simulink model "open_loop"  (R2021b)
settings: Solver=VariableStepAuto  StartTime=0.0  StopTime=100.0  RelTol=1e-3
values from neighbouring files (symbols this model uses):
  A = zeros(size(B'))    [parameters.m]
  I = 4000*eye(3)    [parameters.m]
  Iz = I(end)    [particle_mpc.m]
  m = length(arch_type)    [batch_simulation.m]    (also in particle_mpc.m = mass)
  mass = 2000    [parameters.m]
  r_1 = [front_length;width/2;-height]    [parameters.m]
  radius = 0.4    [parameters.m]
  rear_length = 1.6    [parameters.m]
  sys_d = c2d(sys, ts)    [particle_mpc.m]
  ts = 0.5    [particle_mpc.m]
libraries: nesl_utility x9, autolibshared x5, vrlib x4, mpclib x1
(part 4 of 4)

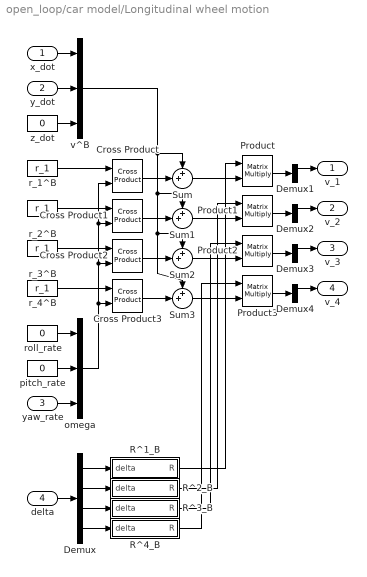
== system open_loop/car model/Longitudinal wheel motion ==
  x_dot : Inport
  y_dot : Inport  Port=2
  yaw_rate : Inport  Port=3
  delta : Inport  Port=4
  Cross Product{,1..3} (4 alike) : vrlib/Utilities/Cross Product
  Demux : Demux
  Demux{1..4} (4 alike) : Demux  Outputs=3
  Product{,1..3} (4 alike) : Product  Multiplication=Matrix(*)
  R^1_B : MATLAB Function  TreatAsAtomicUnit=on
  R^2_B : MATLAB Function  TreatAsAtomicUnit=on
  R^3_B : MATLAB Function  TreatAsAtomicUnit=on
  R^4_B : MATLAB Function  TreatAsAtomicUnit=on
  Sum{,1..3} (4 alike) : Sum  Inputs=++|
  omega : Mux  Inputs=3
  pitch_rate : Constant  Value=0
  r_1^B : Constant  Value=r_1
  r_2^B : Constant  Value=r_1
  r_3^B : Constant  Value=r_1
  r_4^B : Constant  Value=r_1
  roll_rate : Constant  Value=0
  v^B : Mux  Inputs=3
  z_dot : Constant  Value=0
  v_1 : Outport
  v_2 : Outport  Port=2
  v_3 : Outport  Port=3
  v_4 : Outport  Port=4
  wires:
  x_dot/1 -> v^B/1
  y_dot/1 -> v^B/2
  z_dot/1 -> v^B/3
  yaw_rate/1 -> omega/3
  roll_rate/1 -> omega/1
  pitch_rate/1 -> omega/2
  r_1^B/1 -> Cross Product/1
  omega/1 -> Cross Product3/2, Cross Product2/2, Cross Product/2, Cross Product1/2
  r_2^B/1 -> Cross Product1/1
  r_3^B/1 -> Cross Product2/1
  r_4^B/1 -> Cross Product3/1
  Cross Product/1 -> Sum/2
  Cross Product1/1 -> Sum1/2
  Cross Product2/1 -> Sum2/2
  Cross Product3/1 -> Sum3/2
  v^B/1 -> Sum/1, Sum1/1, Sum2/1, Sum3/1
  delta/1 -> Demux/1
  Demux/1 -> R^1_B/1(delta)
  Demux/2 -> R^2_B/1(delta)
  Demux/3 -> R^3_B/1(delta)
  Demux/4 -> R^4_B/1(delta)
  Sum/1 -> Product/2
  Sum1/1 -> Product1/2
  Sum2/1 -> Product2/2
  Sum3/1 -> Product3/2
  R^1_B/1(R) -> Product/1
  R^2_B/1(R) -> Product1/1
  R^3_B/1(R) -> Product2/1
  R^4_B/1(R) -> Product3/1
  Product/1 -> Demux1/1
  Demux1/1 -> v_1/1
  Demux2/1 -> v_2/1
  Demux3/1 -> v_3/1
  Demux4/1 -> v_4/1
  Product3/1 -> Demux4/1
  Product1/1 -> Demux2/1
  Product2/1 -> Demux3/1

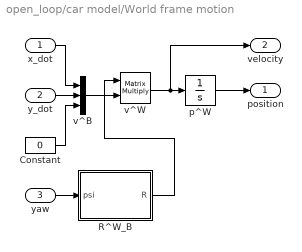
== system open_loop/car model/World frame motion ==
  x_dot : Inport
  y_dot : Inport  Port=2
  yaw : Inport  Port=3
  Constant : Constant  Value=0
  R^W_B : MATLAB Function  TreatAsAtomicUnit=on
  p^W : Integrator
  v^B : Mux  Inputs=3
  v^W : Product  Multiplication=Matrix(*)
  position : Outport
  velocity : Outport  Port=2
  wires:
  yaw/1 -> R^W_B/1(psi)
  y_dot/1 -> v^B/2
  x_dot/1 -> v^B/1
  Constant/1 -> v^B/3
  v^B/1 -> v^W/2
  R^W_B/1(R) -> v^W/1
  v^W/1 -> velocity/1, p^W/1
  p^W/1 -> position/1

== matlab function open_loop/car model/Longitudinal wheel motion/R^1_B ==
  data: delta input; R output
function R = wheel_rotation(delta)
R=[cos(delta) sin(delta) 0
  -sin(delta) cos(delta) 0
  0 0 1];

== matlab function open_loop/MPC/MATLAB Function ==
  data: u input; state input; output input; B output; X output; Y output; U output; DX output; m input; Iz input; Ts input
function [B, X, Y, U, DX] = fcn(u, state, output, m, Iz, Ts)
    A_c = [0 0 0 1 0 0;
     0 0 0 0 1 0;
     0 0 0 0 0 1;
     0 0 0 0 0 0;
     0 0 0 0 0 0;
     0 0 0 0 0 0];
    B = [zeros(3,3); 
          [cos(output(3))/m -sin(output(3))/m 0;
           sin(output(3))/m  cos(output(3))/m 0;
           0          0         1/Iz]];

    B = B*Ts; % zero order hold discretization
    X = state;
    Y = output;
    U = u;
    DX = A_c*Ts*state + B*U;
    DX = reshape(DX, [6 1]);
end

== matlab function open_loop/car model/Longitudinal wheel motion/R^2_B ==
  data: delta input; R output
function R = wheel_rotation(delta)
R=[cos(delta) sin(delta) 0
  -sin(delta) cos(delta) 0
  0 0 1];

== matlab function open_loop/car model/Longitudinal wheel motion/R^3_B ==
  data: delta input; R output
function R = wheel_rotation(delta)
R=[cos(delta) sin(delta) 0
  -sin(delta) cos(delta) 0
  0 0 1];

== matlab function open_loop/car model/Longitudinal wheel motion/R^4_B ==
  data: delta input; R output
function R = wheel_rotation(delta)
R=[cos(delta) sin(delta) 0
  -sin(delta) cos(delta) 0
  0 0 1];

== matlab function open_loop/car model/World frame motion/R^W_B ==
  data: psi input; R output
function R = rotation_matrix(psi)
R = [cos(psi) -sin(psi) 0
     sin(psi)  sin(psi) 0
     0         0        1];

== matlab function open_loop/steering angles ==
  data: u input; y output
function y = fcn(u)
min=-pi/2; max=pi/2;
y=mod(u-min,max-min)+min;
